simulink model "QubeServoSimSK"  (R2022a)
settings: Solver=ode4  StartTime=0.0  StopTime=Tsim  FixedStep=Tin  RelTol=1e-3
values from neighbouring files (symbols this model uses):
  CloseLoopFlag = 0    [QubeServoSim.m]
  StudentID = 00    (= 0)    [QubeServoSim.m]
  Tin = 0.1e-3    (= 0.0001)    [QubeServoSim.m]
undefined symbols (not defined in the file or in its folder): Distrubance, Disturbance, Proceso
libraries: simulink x3
settings Model: Creator=Andres Molano  LastModifiedBy=andre
settings SolverCC: AlgebraicLoopSolver=TrustRegion
settings DataIOCC: LimitDataPoints=on  SaveFormat=Array  ReturnWorkspaceOutputs=off
settings OptimizationCC: LifeSpan=inf
settings DebuggingCC: SolverPrmCheckMsg=warning  UnconnectedInputMsg=warning  UnconnectedOutputMsg=warning  UnconnectedLineMsg=warning  SFUnexpectedBacktrackingDiag=warning  SFNoUnconditionalDefaultTransitionDiag=warning  SFExecutionAtInitializationDiag=none  SFMachineParentedDataDiag=warning  ArithmeticOperatorsInVariantConditions=warning
settings HardwareCC: ProdBitPerPointer=32  ProdBitPerSizeT=32  ProdBitPerPtrDiffT=32  ProdLargestAtomicFloat=None  ProdIntDivRoundTo=Undefined  ProdEndianess=Unspecified  ProdWordSize=32  ProdHWDeviceType=32-bit Generic
settings ModelReferenceCC: PropagateSignalLabelsOutOfModel=off
settings SFSimCC: SimUseLocalCustomCode=off  CustomCodeUndefinedFunction=UseInterfaceOnly
settings RTWCC: RTWUseLocalCustomCode=off
settings CodeAppCC: StateflowObjectComments=on
settings GRTTargetCC: TargetLangStandard=C89/C90 (ANSI)
settings ConfigComp: CovMetricSettings=dw  CovSaveCumulativeToWorkspaceVar=on  CovSaveSingleToWorkspaceVar=on  CovExternalEMLEnable=off  CovSFcnEnable=off

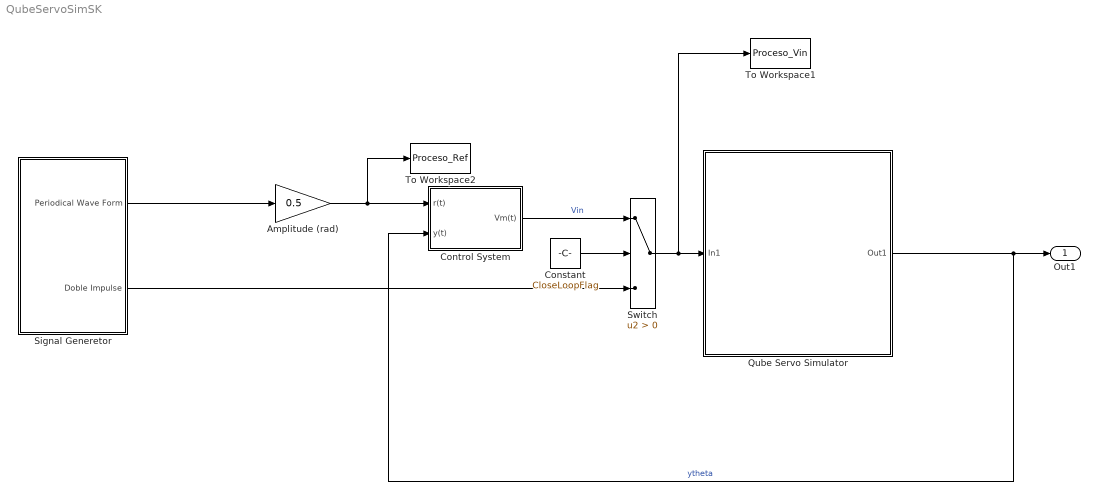
== system QubeServoSimSK ==
  Amplitude (rad) : Gain  Gain=0.5
  Constant : Constant  Value=CloseLoopFlag
  Control System : Subsystem
  Qube Servo Simulator : Subsystem
      mask Display: image('QubeServo.png')
  Signal Generetor : Subsystem
  Switch : Switch  Criteria=u2 > Threshold  SaturateOnIntegerOverflow=off  InputSameDT=off
  To Workspace1 : ToWorkspace  VariableName=Proceso_Vin  SaveFormat=Structure With Time  SampleTime=-1
  To Workspace2 : ToWorkspace  VariableName=Proceso_Ref  SaveFormat=Structure With Time  SampleTime=-1
  Out1 : Outport
  wires:
  Amplitude (rad)/1 -> To Workspace2/1, Control System/1(r(t))
  Qube Servo Simulator/1(Out1) -> Control System/2(y(t)), Out1/1  "ytheta"
  Switch/1 -> To Workspace1/1, Qube Servo Simulator/1(In1)
  Signal Generetor/1(Periodical Wave Form) -> Amplitude (rad)/1
  Constant/1 -> Switch/2
  Control System/1(Vm(t)) -> Switch/1  "Vin"
  Signal Generetor/2(Doble Impulse) -> Switch/3

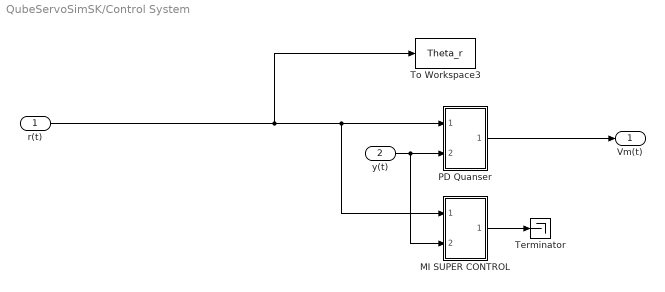
== system QubeServoSimSK/Control System ==
  r(t) : Inport
  y(t) : Inport  Port=2
  MI SUPER CONTROL : Subsystem
  PD Quanser : Subsystem
  Terminator : Terminator
  To Workspace3 : ToWorkspace  VariableName=Theta_r  SaveFormat=Structure With Time  SampleTime=-1
  Vm(t) : Outport
  wires:
  y(t)/1 -> MI SUPER CONTROL/2(y(t)), PD Quanser/2(y(t))
  r(t)/1 -> To Workspace3/1, MI SUPER CONTROL/1(r(t)), PD Quanser/1(r(t))
  PD Quanser/1(Vm(t)) -> Vm(t)/1
  MI SUPER CONTROL/1(Vm(t)) -> Terminator/1

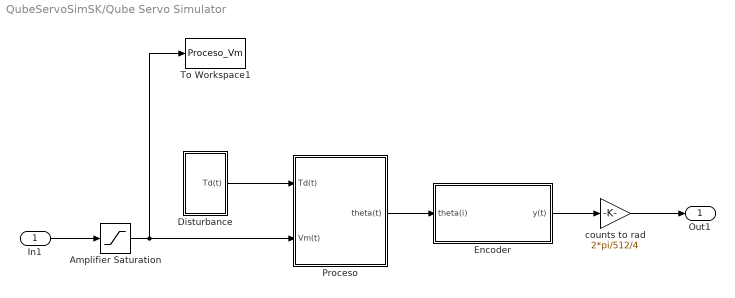
== system QubeServoSimSK/Qube Servo Simulator ==
  In1 : Inport
  Amplifier Saturation : Saturate  UpperLimit=Proceso.VinUP  LowerLimit=Proceso.VinDOWN
  "Disturbance " : Subsystem
  Encoder : Subsystem
  Proceso : Subsystem
  To Workspace1 : ToWorkspace  VariableName=Proceso_Vm  SaveFormat=Structure With Time  SampleTime=-1
  counts to rad : Gain  Gain=2*pi/512/4
  Out1 : Outport
  wires:
  Amplifier Saturation/1 -> Proceso/2(Vm(t)), To Workspace1/1
  Proceso/1(theta(t)) -> Encoder/1(theta(i))
  "Disturbance "/1(Td(t)) -> Proceso/1(Td(t))
  In1/1 -> Amplifier Saturation/1
  Encoder/1(y(t)) -> counts to rad/1
  counts to rad/1 -> Out1/1

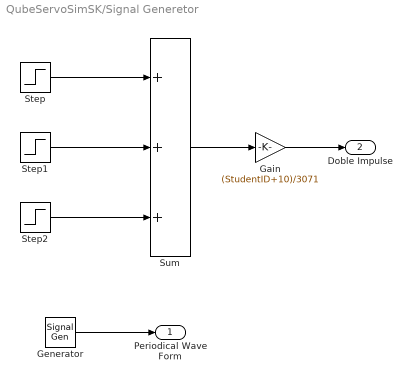
== system QubeServoSimSK/Signal Generetor ==
  Gain : Gain  Gain=(StudentID+10)/3071
  Generator : SignalGenerator  WaveForm=square  Frequency=0.4
  Step : Step  Time=0  SampleTime=0
  Step1 : Step  Time=2  After=-2  SampleTime=0
  Step2 : Step  Time=4  SampleTime=0
  Sum : Sum  Inputs=+++
  Periodical Wave Form : Outport
  Doble Impulse : Outport  Port=2
  wires:
  Generator/1 -> Periodical Wave Form/1
  Sum/1 -> Gain/1
  Step/1 -> Sum/1
  Step1/1 -> Sum/2
  Step2/1 -> Sum/3
  Gain/1 -> Doble Impulse/1

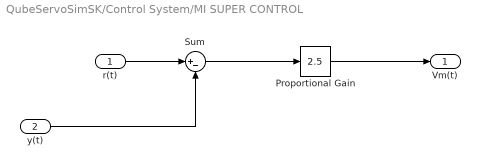
== system QubeServoSimSK/Control System/MI SUPER CONTROL ==
  r(t) : Inport
  y(t) : Inport  Port=2
  Proportional Gain : simulink/Math Operations/Slider Gain  gain=2.5  low=0  high=10
  Sum : Sum  Inputs=|+-
  Vm(t) : Outport
  wires:
  y(t)/1 -> Sum/2
  Sum/1 -> Proportional Gain/1
  r(t)/1 -> Sum/1
  Proportional Gain/1 -> Vm(t)/1

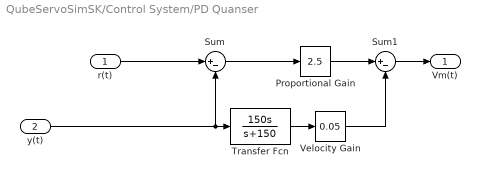
== system QubeServoSimSK/Control System/PD Quanser ==
  r(t) : Inport
  y(t) : Inport  Port=2
  Proportional Gain : simulink/Math Operations/Slider Gain  gain=2.5  low=0  high=10
  Sum : Sum  Inputs=|+-
  Sum1 : Sum  Inputs=|+-
  Transfer Fcn : TransferFcn  Numerator=[150 0]  Denominator=[1 150]
  Velocity Gain : simulink/Math Operations/Slider Gain  gain=0.05  low=0  high=0.5
  Vm(t) : Outport
  wires:
  Sum1/1 -> Vm(t)/1
  Velocity Gain/1 -> Sum1/2
  Transfer Fcn/1 -> Velocity Gain/1
  Proportional Gain/1 -> Sum1/1
  r(t)/1 -> Sum/1
  Sum/1 -> Proportional Gain/1
  y(t)/1 -> Sum/2, Transfer Fcn/1

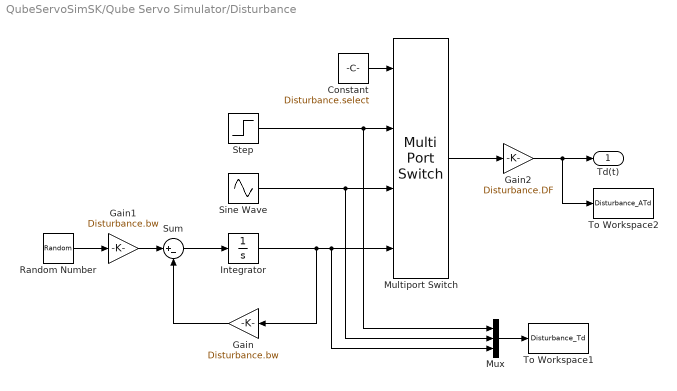
== system QubeServoSimSK/Qube Servo Simulator/Disturbance  ==
  Constant : Constant  Value=Disturbance.select
  Gain : Gain  Gain=Disturbance.bw
  Gain1 : Gain  Gain=Disturbance.bw
  Gain2 : Gain  Gain=Disturbance.DF
  Integrator : Integrator
  Multiport Switch : MultiPortSwitch  DataPortOrder=Zero-based contiguous  zeroidx=on  SaturateOnIntegerOverflow=off  InputSameDT=off
  Mux : Mux  Inputs=3
  Random Number : RandomNumber  Mean=Disturbance.Forder.mean  Variance=Disturbance.Forder.std  Seed=Disturbance.Forder.Seed  SampleTime=Tin
  Sine Wave : Sin  Amplitude=Disturbance.sin.amplitude  Bias=Disturbance.sin.bias  Frequency=Distrubance.sin.omg  SampleTime=Tin
  Step : Step  Time=Disturbance.step.time  Before=Disturbance.step.initialvalue  After=Disturbance.step.finalvalue  SampleTime=Tin
  Sum : Sum  Inputs=|+-
  To Workspace1 : ToWorkspace  VariableName=Disturbance_Td  SaveFormat=Structure With Time  SampleTime=-1
  To Workspace2 : ToWorkspace  VariableName=Disturbance_ATd  SaveFormat=Structure With Time  SampleTime=-1
  Td(t) : Outport
  wires:
  Gain1/1 -> Sum/1
  Sum/1 -> Integrator/1
  Integrator/1 -> Gain/1, Mux/3, Multiport Switch/4
  Gain/1 -> Sum/2
  Constant/1 -> Multiport Switch/1
  Sine Wave/1 -> Mux/2, Multiport Switch/3
  Multiport Switch/1 -> Gain2/1
  Step/1 -> Mux/1, Multiport Switch/2
  Random Number/1 -> Gain1/1
  Gain2/1 -> To Workspace2/1, Td(t)/1
  Mux/1 -> To Workspace1/1

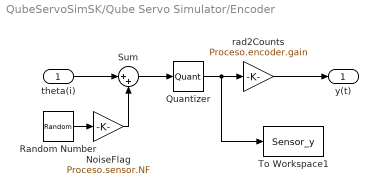
== system QubeServoSimSK/Qube Servo Simulator/Encoder ==
  theta(i) : Inport
  NoiseFlag : Gain  Gain=Proceso.sensor.NF
  Quantizer : Quantizer  QuantizationInterval=Proceso.encoder.dQ
  Random Number : RandomNumber  Mean=Proceso.sensor.error.mean  Variance=Proceso.sensor.error.std^2  Seed=Proceso.sensor.error.seed  SampleTime=Tin
  Sum : Sum  Inputs=|++
  To Workspace1 : ToWorkspace  VariableName=Sensor_y  SaveFormat=Structure With Time  SampleTime=-1
  rad2Counts : Gain  Gain=Proceso.encoder.gain
  y(t) : Outport
  wires:
  Quantizer/1 -> To Workspace1/1, rad2Counts/1
  rad2Counts/1 -> y(t)/1
  theta(i)/1 -> Sum/1
  Sum/1 -> Quantizer/1
  Random Number/1 -> NoiseFlag/1
  NoiseFlag/1 -> Sum/2

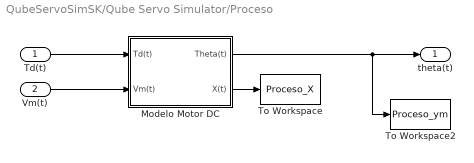
== system QubeServoSimSK/Qube Servo Simulator/Proceso ==
  Td(t) : Inport
  Vm(t) : Inport  Port=2
  Modelo Motor DC : Subsystem
  To Workspace : ToWorkspace  VariableName=Proceso_X  SaveFormat=Structure With Time  SampleTime=-1
  To Workspace2 : ToWorkspace  VariableName=Proceso_ym  SaveFormat=Structure With Time  SampleTime=-1
  theta(t) : Outport
  wires:
  Modelo Motor DC/2(X(t)) -> To Workspace/1
  Td(t)/1 -> Modelo Motor DC/1(Td(t))
  Vm(t)/1 -> Modelo Motor DC/2(Vm(t))
  Modelo Motor DC/1(Theta(t)) -> To Workspace2/1, theta(t)/1

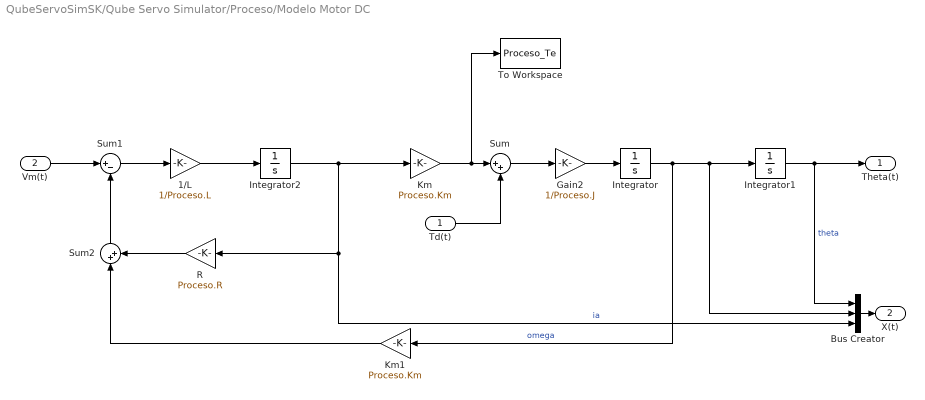
== system QubeServoSimSK/Qube Servo Simulator/Proceso/Modelo Motor DC ==
  Td(t) : Inport
  Vm(t) : Inport  Port=2
  1/L : Gain  Gain=1/Proceso.L
  Bus Creator : BusCreator  Inputs=3
  Gain2 : Gain  Gain=1/Proceso.J
  Integrator : Integrator  InitialCondition=Proceso.X0.omg
  Integrator1 : Integrator  InitialCondition=Proceso.X0.theta
  Integrator2 : Integrator  InitialCondition=Proceso.X0.im
  Km : Gain  Gain=Proceso.Km
  Km1 : Gain  Gain=Proceso.Km
  R : Gain  Gain=Proceso.R
  Sum : Sum  Inputs=|++
  Sum1 : Sum  Inputs=|+-
  Sum2 : Sum  Inputs=|++
  To Workspace : ToWorkspace  VariableName=Proceso_Te  SaveFormat=Structure With Time  SampleTime=-1
  Theta(t) : Outport
  X(t) : Outport  Port=2
  wires:
  Sum1/1 -> 1/L/1
  Integrator/1 -> Bus Creator/2, Integrator1/1, Km1/1  "omega"
  Km/1 -> To Workspace/1, Sum/1
  R/1 -> Sum2/2
  Gain2/1 -> Integrator/1
  Integrator2/1 -> Bus Creator/3, R/1, Km/1  "ia"
  Sum/1 -> Gain2/1
  1/L/1 -> Integrator2/1
  Sum2/1 -> Sum1/2
  Td(t)/1 -> Sum/2
  Vm(t)/1 -> Sum1/1
  Integrator1/1 -> Bus Creator/1, Theta(t)/1  "theta"
  Km1/1 -> Sum2/1
  Bus Creator/1 -> X(t)/1
